simulink model "board_algorithm_2note_length"  (R2023b)
settings: Solver=FixedStepAuto  StartTime=0.0  StopTime=100000.0  RelTol=1e-3
values from neighbouring files (symbols this model uses):
  f_s = 11025    [main.m]
  in_table = single([[0],excitation])    [main.m]
  input = midiMsg_to_input(msgArray)    [main.m]
  N_n = floor(f_s/bps)    [main.m]
  period_sequence_1 = [normalised_period(f_s,input_seq_1(1,:)) ... (first row only)    [main.m]
  period_sequence_2 = [normalised_period(f_s,input_seq_2(1,:)) ... (first row only)    [main.m]
  seq_length = length(input_seq_1)+1    [main.m]
undefined symbols (not defined in the file or in its folder): frac_delay_inter, GPTRIP1SEL, GPTRIP2SEL, TZ1, TZ2
libraries: tiiqmathlib x8, simulink x5, c2837xDlib x3, dspindex x2, c2000lib x1, c280xlib x1, c2802xlib x1
settings Model: ExtModeTrigDuration=8  Creator=andre  LastModifiedBy=Rorya
settings OptimizationCC: DefaultUnderspecifiedDataType=single  EnhancedBackFolding=on  PassReuseOutputArgsAs=Individual arguments  MaxStackSize=1024  OptimizeBlockOrder=speed  DifferentSizesBufferReuse=on  OptimizationCustomize=off  EfficientTunableParamExpr=on
settings DebuggingCC: ParameterTunabilityLossMsg=error
settings HardwareCC: ProdBitPerChar=16  ProdBitPerInt=16  ProdBitPerPointer=32  ProdBitPerSizeT=32  ProdBitPerPtrDiffT=32  ProdLargestAtomicInteger=Integer  ProdLargestAtomicFloat=None  ProdWordSize=16  ProdLongLongMode=on  ProdHWDeviceType=Texas Instruments->C2000  HardwareBoardFeatureSet=SoCBlockset
settings ModelReferenceCC: ModelReferenceNumInstancesAllowed=Single
settings SFSimCC: MATLABDynamicMemAlloc=off
settings RTWCC: Description=Embedded Coder  SystemTargetFile=ert.tlc  HardwareBoard=TI Delfino F28379D LaunchPad  TemplateMakefile=ert_default_tmf  GenerateReport=on  Toolchain=Texas Instruments Code Composer Studio (C2000)  LaunchReport=on  CodeExecutionProfiling=on  CodeProfilingSaveOptions=AllData  CodeProfilingInstrumentation=detailed
settings CodeAppCC: ForceParamTrailComments=on  IgnoreCustomStorageClasses=off  OperatorAnnotations=on  SimulinkDataObjDesc=on  SFDataObjDesc=on  InsertBlockDesc=on
settings ERTTargetCC: CodeReplacementLibrary=TI C28x  ExtModeTransport=4  ExtModeStaticAlloc=on  ExtModeAutomaticAllocSize=off  ExtModeStaticAllocSize=10000  ExtModeMexFile=ext_xcp  ExtModeIntrfLevel=Level2 - Open

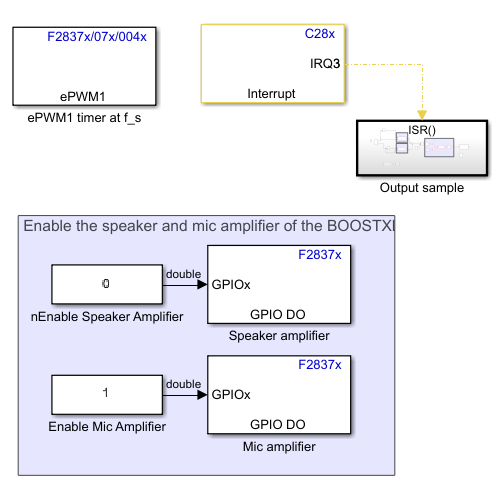
[thumbnail: Simulink's stored preview of the top-level diagram]
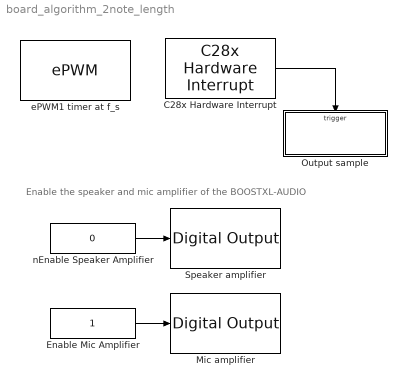
== system board_algorithm_2note_length ==
  note: Enable the speaker and mic amplifier of the BOOSTXL-AUDIO
  C28x Hardware Interrupt : c2000lib/Scheduling/C28x Hardware Interrupt  irqnumbers=[3]  pienumbers=[1]  irqpriorities=[30]  irqpreempts=[1]  showinput=off  dspchiptype=C280X
  Enable Mic Amplifier : Constant
  Mic amplifier : c2837xDlib/Digital Output  GPIO_Number=GPIO96~GPIO103  GPIO_Bit0=off  GPIO_BIT0_Toggle=off  GPIO_Bit1=on  GPIO_BIT1_Toggle=off  GPIO_Bit2=off  GPIO_BIT2_Toggle=off  GPIO_Bit3=off  GPIO_BIT3_Toggle=off  GPIO_Bit4=off  GPIO_BIT4_Toggle=off  GPIO_Bit5=off  GPIO_BIT5_Toggle=off  GPIO_Bit6=off  GPIO_BIT6_Toggle=off  GPIO_Bit7=off  GPIO_BIT7_Toggle=off
  Output sample : Subsystem  TreatAsAtomicUnit=on
  Speaker amplifier : c2837xDlib/Digital Output  GPIO_Number=GPIO24~GPIO31  GPIO_Bit0=off  GPIO_BIT0_Toggle=off  GPIO_Bit1=off  GPIO_BIT1_Toggle=off  GPIO_Bit2=on  GPIO_BIT2_Toggle=off  GPIO_Bit3=off  GPIO_BIT3_Toggle=off  GPIO_Bit4=off  GPIO_BIT4_Toggle=off  GPIO_Bit5=off  GPIO_BIT5_Toggle=off  GPIO_Bit6=off  GPIO_BIT6_Toggle=off  GPIO_Bit7=off  GPIO_BIT7_Toggle=off
  ePWM1 timer at f_s : c2802xlib/ePWM  PwmType=C2000_Type4  useModule=ePWM1  ePWMxLINKTBPRD=Not Linked  periodUnits=Seconds  timerSource=Specify via dialog  timerPeriod_clk=1000  timerPeriod_sec=1/f_s  tbshadow=Counter equals to zero  countingMode=Up  phaseActiveEnable=Set counter to phase value specified via dialog  phaseDirection=Count down after sync  phaseActive=6250  synchronizationEnable=off  dcaevt1Sync=off  dcbevt1Sync=off  synchronizationOption=Disable  dcbevt1SyncOut=off  dcaevt1SyncOut=off  cmpdSyncOut=off  cmpcSyncOut=off  cmpbSyncOut=off  zeroSyncOut=off  swfSyncOut=off  perSynchronizationOption=Counter equals to period (CTR=PRD)  clockPrescale=1  HSclockPrescale=1  enswap=off  ePWMxAStatus=off  ePWMxAactionLogic1=Do nothing  ePWMxAactionLogic2=Do nothing  ePWMxAactionLogic3=Do nothing  ePWMxAactionLogic4=Set  ePWMxAactionLogic5=Do nothing  ePWMxAactionLogic6=Do nothing  ePWMxACSFenable=off  ePWMxACSFvalue=Forcing disable  ePWMxASFreload=Zero  ePWMxBStatus=off  ePWMxBactionLogic1=Set  ePWMxBactionLogic2=Clear  ePWMxBactionLogic3=Do nothing  ePWMxBactionLogic4=Do nothing  ePWMxBactionLogic5=Clear  ePWMxBactionLogic6=Set  ePWMxBCSFenable=off  ePWMxBCSFvalue=Forcing disable  ePWMxBSFreload=Zero  ePWNxBOutWay=off  ePWMxLINKCMPA=Not Linked  CMPAUnits=Percentages  CMPASource=Specify via dialog  CMPAValue_per=50  CMPAValue_clk=50  enCMPAshadow=Counter equals to zero (CTR=Zero)  ePWMxLINKCMPB=Not Linked  CMPBUnits=Clock cycles  CMPBSource=Specify via dialog  CMPBValue_per=50  CMPBValue_clk=32000  enCMPBshadow=Counter equals to zero (CTR=Zero)  ePWMxLINKCMPC=Not Linked  CMPCUnits=Clock cycles  CMPCSource=Specify via dialog  CMPCValue_per=50  CMPCValue_clk=32000  enCMPCshadow=Counter equals to zero (CTR=Zero)  ePWMxLINKCMPD=Not Linked  CMPDUnits=Clock cycles  CMPDSource=Specify via dialog  CMPDValue_per=50  CMPDValue_clk=32000  enCMPDshadow=Counter equals to zero (CTR=Zero)  enableDBePWMxA=off  enableDBePWMxB=off  enhalfcycle=off  DBpolarity=Active high (AH)  DBedgeDelay=Positive  DBSource_ePWMxA=ePWMxA  DBSource_ePWMxB=ePWMxA  DBPeriodUnits=Clock cycles  DBperiodSource=Specify via dialog  REDperiod=0  FEDperiod=0  REDperiod_sec=0  FEDperiod_sec=0  LoadModeDBRED=Immediate without using shadow  LoadModeDBFED=Immediate without using shadow  adcstartModuleA=off  adcrequestEventA=First event  adcstartEventA=Digital Compare Module A Event 1 start of conversion (DCAEVT1.soc)  adcstartEventA_type2=Counter equals to zero (CTR=Zero)  adcstartModuleB=off  adcrequestEventB=First event  adcstartEventB=Counter equals to zero (CTR=Zero)  adcstartEventB_type2=Counter equals to zero (CTR=Zero)  intEn=on  intPrd=First event  intSel=Counter equals to zero (CTR=Zero)  intSel_type2=Counter equals to zero (CTR=Zero)  hrpe=off  enHRPWM=off  HRPWM_LoadMode=Counter equals to period (CTR=PRD)  HRPWM_CTLMode=Duty or Period control mode  HRPWM_EDGMode=Both edge  hrpeb=off  enHRPWMB=off  HRPWM_LoadModeB=Counter equals to zero (CTR=ZERO)  HRPWM_CTLModeB=Duty or Period control mode  HRPWM_EDGModeB=Both edge  enHRDBRED=off  enHRDBFED=off  enSFO=on  enautoconv=on  chopperEnable=off  chopperFrequency=1  chopperFirstwidth=1  chopperDuty=12.5%  tripZonesource=Specify via dialog  tzselOSHT1=off  tzselOSHT2=off  tzselOSHT3=off  tzselOSHDCAEV1=off  tzselOSHDCBEV1=off  tzselCBC1=off  tzselCBC2=off  tzselCBC3=off  tzselCBCDCAEV2=off  tzselCBCDCBEV2=off  tzselOSHT4=off  tzselOSHT5=off  tzselOSHT6=off  tzselCBC4=off  tzselCBC5=off  tzselCBC6=off  enTzOstIntr=off  enTzCbcIntr=off  enTzDCAEVT1Intr=off  enTzDCAEVT2Intr=off  enTzDCBEVT1Intr=off  enTzDCBEVT2Intr=off  ePWMxAforced=No action  ePWMxBforced=No action  DCAEVT1forced=No action  DCBEVT1forced=No action  DCAEVT2forced=No action  DCBEVT2forced=No action  dcah=Trip Zone 1 input (TZ1)  dcal=Trip Zone 2 input (TZ2)  dcbh=Trip Zone 1 input (TZ1)  dcbl=Trip Zone 2 input (TZ2)  dcah_type2=GPTRIP1SEL/(TZ1)  dcal_type2=GPTRIP2SEL/(TZ2)  dcbh_type2=GPTRIP1SEL/(TZ1)  dcbl_type2=GPTRIP2SEL/(TZ2)  gendcaevt1=Event disabled  gendcaevt2=Event disabled  gendcbevt1=Event disabled  gendcbevt2=Event disabled  dcaevt1src=DCAEVT1 with sync  dcaevt2src=DCAEVT2 with sync  dcbevt1src=DCBEVT1 with sync  dcbevt2src=DCBEVT2 with sync  pulsesel=Counter equals to zero (CTR=Zero)  blankinv=off  blankoffset=0  blankwidth=0  evsrcsel=Filtered version of DCAEVT1 (DCAEVT1FILT)  encape=off
  nEnable Speaker Amplifier : Constant  Value=0
  wires:
  Enable Mic Amplifier/1 -> Mic amplifier/1
  nEnable Speaker Amplifier/1 -> Speaker amplifier/1
  C28x Hardware Interrupt/1 -> Output sample/Trigger

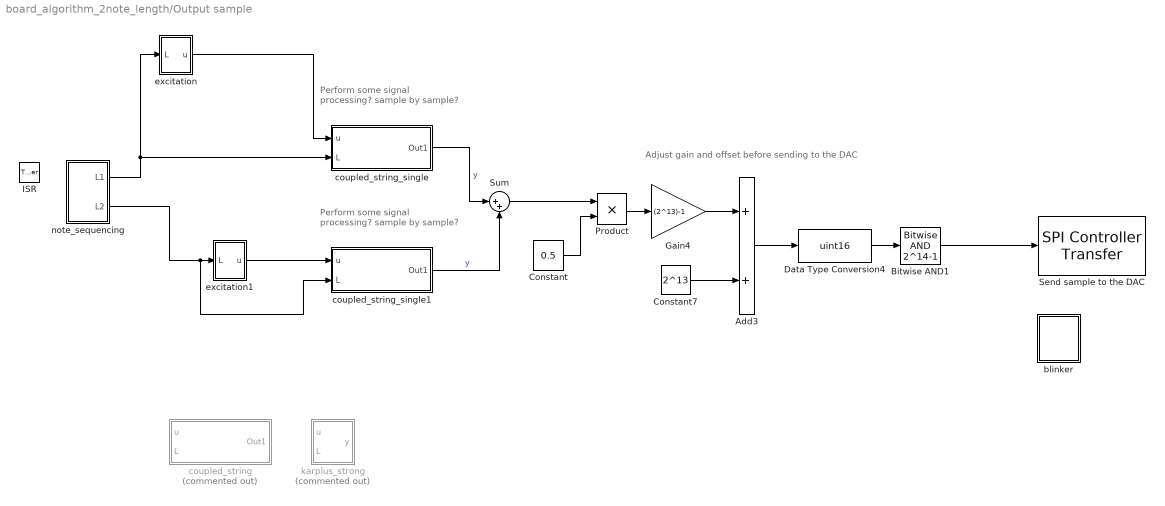
== system board_algorithm_2note_length/Output sample ==
  note: Adjust gain and offset before sending to the DAC
  note: Perform some signal
      | processing?
      | sample by sample?
  note: Perform some signal
      | processing?
      | sample by sample?
  ISR : TriggerPort  TriggerType=function-call  VariantControl=(inherit)
  Add3 : Sum
  Bitwise AND1 : simulink/Logic and Bit Operations/Bitwise Operator  logicop=AND  UseBitMask=on  BitMask=2^14-1  BitMaskRealWorld=Stored Integer
  Constant : Constant  Value=0.5
  Constant7 : Constant  Value=2^13  OutDataTypeStr=single
  Data Type Conversion4 : DataTypeConversion  OutDataTypeStr=uint16  SaturateOnIntegerOverflow=off  RndMeth=Floor
  Gain4 : Gain  Gain=(2^13)-1
  Product : Product
  Send sample to the DAC : c280xlib/SPI Controller Transfer  SPISelect=SPI_B  ClockPolarity=Rising_edge  ClockPhase=Delay_half_cycle  SPIModule=uint32(0)  Mode=Master  BusSpeed=uint32(1000000)  FirstBitToTransfer=Most significant bit (MSB)  ClockMode=0  BlockFunction=Transfer  EnableRegisterAddress=off  RegisterAddress=0  OutputDataType=int8  OutputDataLength=1  DataBits=16  UseCustomSSPin=Explicit GPIO calls  ActiveLowSSPin=Active low  Pin=27
  Sum : Sum  Inputs=|++
  blinker : Subsystem
  coupled_string : Subsystem  Commented=on
  coupled_string_single : Subsystem
  coupled_string_single1 : Subsystem
  excitation : Subsystem
  excitation1 : Subsystem
  karplus_strong : Subsystem  Commented=on
  note_sequencing : Subsystem
  wires:
  Data Type Conversion4/1 -> Bitwise AND1/1
  Gain4/1 -> Add3/1
  Bitwise AND1/1 -> Send sample to the DAC/1
  Add3/1 -> Data Type Conversion4/1
  Constant7/1 -> Add3/2
  coupled_string_single/1(Out1) -> Sum/1  "y"
  coupled_string_single1/1(Out1) -> Sum/2  "y"
  Sum/1 -> Product/1
  Constant/1 -> Product/2
  note_sequencing/2(L2) -> coupled_string_single1/2(L), excitation1/1(L)
  Product/1 -> Gain4/1
  excitation/1(u) -> coupled_string_single/1(u)
  note_sequencing/1(L1) -> coupled_string_single/2(L), excitation/1(L)
  excitation1/1(u) -> coupled_string_single1/1(u)

== system board_algorithm_2note_length/Output sample/blinker ==
  Add : Sum
  Blink LED : c2837xDlib/Digital Output  GPIO_Number=GPIO24~GPIO31  GPIO_Bit0=off  GPIO_BIT0_Toggle=off  GPIO_Bit1=off  GPIO_BIT1_Toggle=off  GPIO_Bit2=off  GPIO_BIT2_Toggle=off  GPIO_Bit3=off  GPIO_BIT3_Toggle=off  GPIO_Bit4=off  GPIO_BIT4_Toggle=off  GPIO_Bit5=off  GPIO_BIT5_Toggle=off  GPIO_Bit6=off  GPIO_BIT6_Toggle=off  GPIO_Bit7=on  GPIO_BIT7_Toggle=on
  Compare To Zero : simulink/Logic and Bit Operations/Compare To Zero  relop===  OutDataTypeStr=uint8
  Constant1 : Constant  OutDataTypeStr=uint16
  Constant2 : Constant  Value=f_s  OutDataTypeStr=uint16
  Mod : Math  Operator=mod
  Unit Delay : UnitDelay  SampleTime=-1  HasFrameUpgradeWarning=on
  wires:
  Compare To Zero/1 -> Blink LED/1
  Mod/1 -> Unit Delay/1, Compare To Zero/1
  Unit Delay/1 -> Add/2
  Add/1 -> Mod/1
  Constant2/1 -> Mod/2
  Constant1/1 -> Add/1

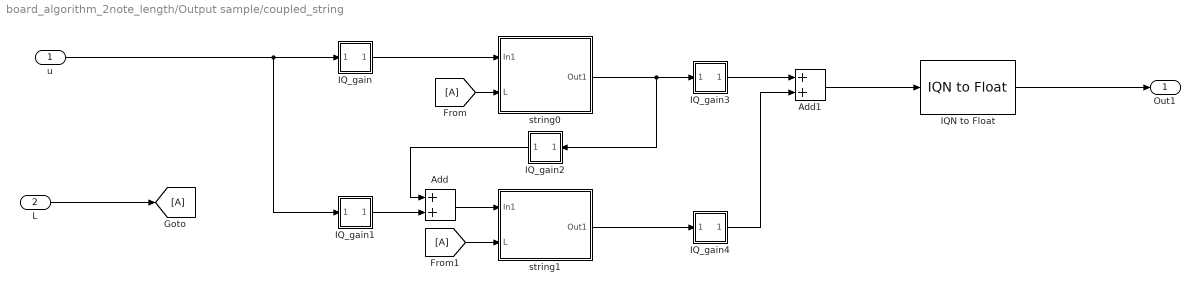
== system board_algorithm_2note_length/Output sample/coupled_string ==
  u : Inport
  L : Inport  Port=2
  Add : Sum  OutDataTypeStr=fixdt(1,32,30)  AccumDataTypeStr=fixdt(1,32,30)
  Add1 : Sum  OutDataTypeStr=Inherit: Same as first input
  From : From
  From1 : From
  Goto : Goto
  IQN to Float : tiiqmathlib/IQN to Float
  IQ_gain : Subsystem
  IQ_gain1 : Subsystem
  IQ_gain2 : Subsystem
  IQ_gain3 : Subsystem
  IQ_gain4 : Subsystem
  string0 : Subsystem
  string1 : Subsystem
  Out1 : Outport
  wires:
  string0/1(Out1) -> IQ_gain3/1(In1), IQ_gain2/1(In1)
  Add/1 -> string1/1(In1)
  IQ_gain/1(Out1) -> string0/1(In1)
  IQ_gain2/1(Out1) -> Add/1
  IQ_gain1/1(Out1) -> Add/2
  string1/1(Out1) -> IQ_gain4/1(In1)
  IQ_gain3/1(Out1) -> Add1/1
  Add1/1 -> IQN to Float/1
  L/1 -> Goto/1
  From/1 -> string0/2(L)
  From1/1 -> string1/2(L)
  IQ_gain4/1(Out1) -> Add1/2
  IQN to Float/1 -> Out1/1
  u/1 -> IQ_gain1/1(In1), IQ_gain/1(In1)

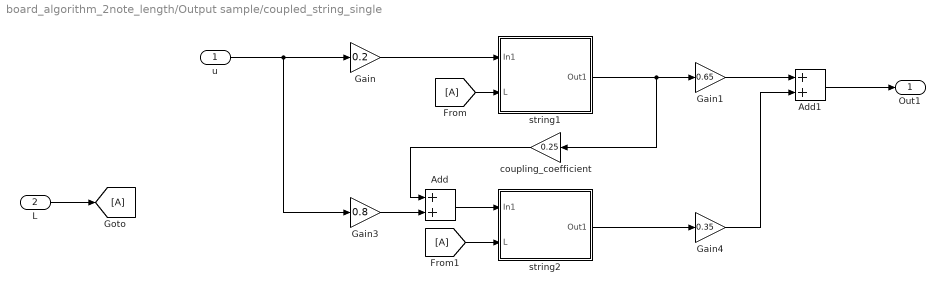
== system board_algorithm_2note_length/Output sample/coupled_string_single ==
  u : Inport  OutDataTypeStr=single
  L : Inport  Port=2
  Add : Sum
  Add1 : Sum
  From : From
  From1 : From
  Gain : Gain  Gain=0.2
  Gain1 : Gain  Gain=0.65
  Gain3 : Gain  Gain=0.8
  Gain4 : Gain  Gain=0.35
  Goto : Goto
  coupling_coefficient : Gain  Gain=0.25
  string1 : Subsystem
  string2 : Subsystem
  Out1 : Outport  OutDataTypeStr=single
  wires:
  string1/1(Out1) -> coupling_coefficient/1, Gain1/1
  Add/1 -> string2/1(In1)
  Gain/1 -> string1/1(In1)
  coupling_coefficient/1 -> Add/1
  Gain3/1 -> Add/2
  string2/1(Out1) -> Gain4/1
  Gain1/1 -> Add1/1
  From/1 -> string1/2(L)
  From1/1 -> string2/2(L)
  Gain4/1 -> Add1/2
  u/1 -> Gain/1, Gain3/1
  L/1 -> Goto/1
  Add1/1 -> Out1/1

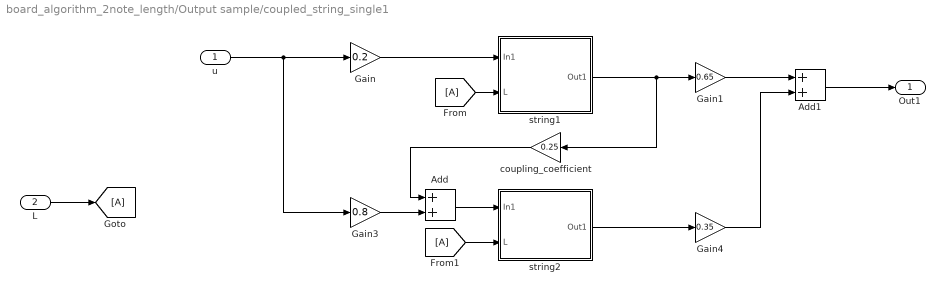
== system board_algorithm_2note_length/Output sample/coupled_string_single1 ==
  u : Inport  OutDataTypeStr=single
  L : Inport  Port=2
  Add : Sum
  Add1 : Sum
  From : From
  From1 : From
  Gain : Gain  Gain=0.2
  Gain1 : Gain  Gain=0.65
  Gain3 : Gain  Gain=0.8
  Gain4 : Gain  Gain=0.35
  Goto : Goto
  coupling_coefficient : Gain  Gain=0.25
  string1 : Subsystem
  string2 : Subsystem
  Out1 : Outport  OutDataTypeStr=single
  wires:
  string1/1(Out1) -> coupling_coefficient/1, Gain1/1
  Add/1 -> string2/1(In1)
  Gain/1 -> string1/1(In1)
  coupling_coefficient/1 -> Add/1
  Gain3/1 -> Add/2
  string2/1(Out1) -> Gain4/1
  Gain1/1 -> Add1/1
  From/1 -> string1/2(L)
  From1/1 -> string2/2(L)
  Gain4/1 -> Add1/2
  u/1 -> Gain/1, Gain3/1
  L/1 -> Goto/1
  Add1/1 -> Out1/1

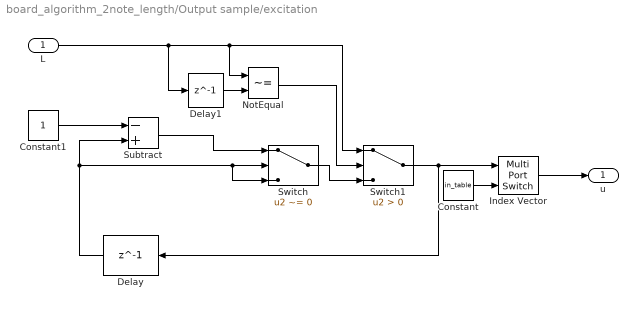
== system board_algorithm_2note_length/Output sample/excitation ==
  L : Inport
  Constant : Constant  Value=in_table  SampleTime=-1
  Constant1 : Constant  SampleTime=-1
  Delay : Delay  DelayLength=1  InitialCondition=0  UseCircularBuffer=on
  Delay1 : Delay  DelayLength=1
  Index Vector : MultiPortSwitch  DataPortOrder=Zero-based contiguous  Inputs=1  zeroidx=on  SaturateOnIntegerOverflow=off  InputSameDT=off
  NotEqual : RelationalOperator  Operator=~=  OutDataTypeStr=boolean  RndMeth=Simplest  InputSameDT=off
  Subtract : Sum  Inputs=-+
  Switch : Switch  Criteria=u2 ~= 0  SaturateOnIntegerOverflow=off  InputSameDT=off
  Switch1 : Switch  Criteria=u2 > Threshold  SaturateOnIntegerOverflow=off  InputSameDT=off
  u : Outport
  wires:
  Constant1/1 -> Subtract/1
  Subtract/1 -> Switch/1
  Switch1/1 -> Index Vector/1, Delay/1
  L/1 -> Delay1/1, NotEqual/1, Switch1/1
  NotEqual/1 -> Switch1/2
  Delay1/1 -> NotEqual/2
  Delay/1 -> Switch/3, Switch/2, Subtract/2
  Switch/1 -> Switch1/3
  Index Vector/1 -> u/1
  Constant/1 -> Index Vector/2

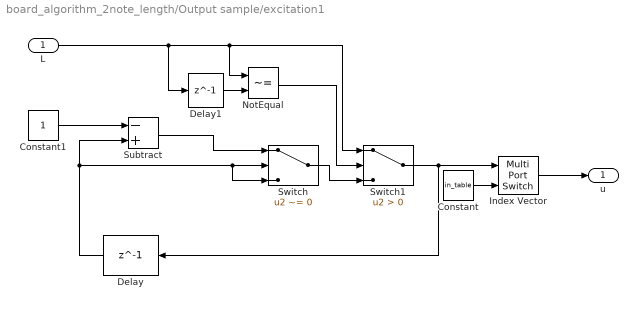
== system board_algorithm_2note_length/Output sample/excitation1 ==
  L : Inport
  Constant : Constant  Value=in_table  SampleTime=-1
  Constant1 : Constant  SampleTime=-1
  Delay : Delay  DelayLength=1  InitialCondition=0  UseCircularBuffer=on
  Delay1 : Delay  DelayLength=1
  Index Vector : MultiPortSwitch  DataPortOrder=Zero-based contiguous  Inputs=1  zeroidx=on  SaturateOnIntegerOverflow=off  InputSameDT=off
  NotEqual : RelationalOperator  Operator=~=  OutDataTypeStr=boolean  RndMeth=Simplest  InputSameDT=off
  Subtract : Sum  Inputs=-+
  Switch : Switch  Criteria=u2 ~= 0  SaturateOnIntegerOverflow=off  InputSameDT=off
  Switch1 : Switch  Criteria=u2 > Threshold  SaturateOnIntegerOverflow=off  InputSameDT=off
  u : Outport
  wires:
  Constant1/1 -> Subtract/1
  Subtract/1 -> Switch/1
  Switch1/1 -> Index Vector/1, Delay/1
  L/1 -> Delay1/1, NotEqual/1, Switch1/1
  NotEqual/1 -> Switch1/2
  Delay1/1 -> NotEqual/2
  Delay/1 -> Switch/3, Switch/2, Subtract/2
  Switch/1 -> Switch1/3
  Index Vector/1 -> u/1
  Constant/1 -> Index Vector/2

== system board_algorithm_2note_length/Output sample/karplus_strong ==
  u : Inport
  L : Inport  Port=2
  Discrete FIR Filter : DiscreteFir
  Sum : Sum  Inputs=|++
  Variable Integer Delay : Delay  DelayLengthSource=Input port  DelayLengthUpperLimit=256  PreventDirectFeedthrough=on  UseCircularBuffer=on
      settings: InputPortMap=u0,p1
  decay constant : Gain
  y : Outport
  wires:
  Variable Integer Delay/1 -> Discrete FIR Filter/1
  L/1 -> Variable Integer Delay/2
  decay constant/1 -> Sum/2
  Sum/1 -> y/1, Variable Integer Delay/1  "y"
  u/1 -> Sum/1
  Discrete FIR Filter/1 -> decay constant/1

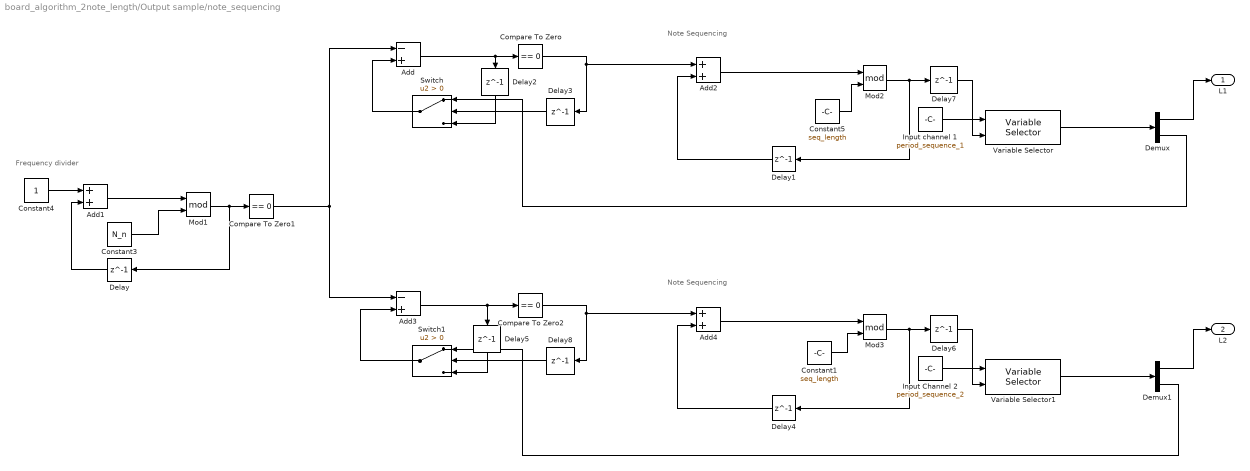
== system board_algorithm_2note_length/Output sample/note_sequencing ==
  note: Frequency divider
  note: Note Sequencing
  note: Note Sequencing
  Add : Sum  Inputs=-+
  Add1 : Sum
  Add2 : Sum
  Add3 : Sum  Inputs=-+
  Add4 : Sum
  Compare To Zero : simulink/Logic and Bit Operations/Compare To Zero  relop===  OutDataTypeStr=boolean
  Compare To Zero1 : simulink/Logic and Bit Operations/Compare To Zero  relop===  OutDataTypeStr=boolean
  Compare To Zero2 : simulink/Logic and Bit Operations/Compare To Zero  relop===  OutDataTypeStr=boolean
  Constant1 : Constant  Value=seq_length  OutDataTypeStr=uint32
  Constant3 : Constant  Value=N_n  OutDataTypeStr=uint32
  Constant4 : Constant  OutDataTypeStr=uint32
  Constant5 : Constant  Value=seq_length  OutDataTypeStr=uint32
  Delay : Delay  DelayLength=1  InitialCondition=0  UseCircularBuffer=on
  Delay1 : Delay  DelayLength=1  InitialCondition=0  UseCircularBuffer=on
  Delay{2..3,5..8} (6 alike) : Delay  DelayLength=1  InitialCondition=0
  Delay4 : Delay  DelayLength=1  InitialCondition=0  UseCircularBuffer=on
  Demux : Demux  Outputs=2
  Demux1 : Demux  Outputs=2
  Input Channel 2 : Constant  Value=period_sequence_2
  Input channel 1 : Constant  Value=period_sequence_1
  Mod1 : Math  Operator=mod
  Mod2 : Math  Operator=mod
  Mod3 : Math  Operator=mod
  Switch : Switch  Criteria=u2 > Threshold  SaturateOnIntegerOverflow=off  InputSameDT=off
  Switch1 : Switch  Criteria=u2 > Threshold  SaturateOnIntegerOverflow=off  InputSameDT=off
  Variable Selector : dspindex/Variable Selector  NumInputs=1  rowsOrCols=Columns  IdxMode=Variable  Elements=[1 3]  ZerOneIdxMode=One-based  errmode=Clip Index  FillMode=on  FillValues=0
  Variable Selector1 : dspindex/Variable Selector  NumInputs=1  rowsOrCols=Columns  IdxMode=Variable  Elements=[1 3]  ZerOneIdxMode=One-based  errmode=Clip Index  FillMode=on  FillValues=0
  L1 : Outport
  L2 : Outport  Port=2
  wires:
  Constant5/1 -> Mod2/2
  Demux/2 -> Switch/1
  Delay/1 -> Add1/2
  Delay1/1 -> Add2/2
  Add2/1 -> Mod2/1
  Compare To Zero/1 -> Delay3/1, Add2/1
  Constant3/1 -> Mod1/2
  Mod1/1 -> Compare To Zero1/1, Delay/1
  Mod2/1 -> Delay7/1, Delay1/1
  Demux/1 -> L1/1
  Add1/1 -> Mod1/1
  Input channel 1/1 -> Variable Selector/1
  Constant4/1 -> Add1/1
  Add/1 -> Compare To Zero/1, Delay2/1
  Add3/1 -> Delay5/1, Compare To Zero2/1
  Input Channel 2/1 -> Variable Selector1/1
  Demux1/1 -> L2/1
  Compare To Zero2/1 -> Delay8/1, Add4/1
  Mod3/1 -> Delay6/1, Delay4/1
  Compare To Zero1/1 -> Add3/1, Add/1
  Delay4/1 -> Add4/2
  Add4/1 -> Mod3/1
  Demux1/2 -> Switch1/1
  Constant1/1 -> Mod3/2
  Delay6/1 -> Variable Selector1/2
  Variable Selector1/1 -> Demux1/1
  Delay7/1 -> Variable Selector/2
  Variable Selector/1 -> Demux/1
  Delay3/1 -> Switch/2
  Delay8/1 -> Switch1/2
  Switch/1 -> Add/2
  Switch1/1 -> Add3/2
  Delay5/1 -> Switch1/3
  Delay2/1 -> Switch/3

== system board_algorithm_2note_length/Output sample/coupled_string/IQ_gain ==
  In1 : Inport  OutDataTypeStr=fixdt(1,32,30)
  Constant : Constant  Value=0.2  OutDataTypeStr=fixdt(1,32,30)
  IQN x IQN : tiiqmathlib/IQN x IQN  multiplyOption=Multiply
  Out1 : Outport  OutDataTypeStr=fixdt(1,32,30)
  wires:
  In1/1 -> IQN x IQN/1
  IQN x IQN/1 -> Out1/1
  Constant/1 -> IQN x IQN/2

== system board_algorithm_2note_length/Output sample/coupled_string/IQ_gain1 ==
  In1 : Inport
  Constant : Constant  Value=0.8  OutDataTypeStr=fixdt(1,32,30)
  IQN x IQN : tiiqmathlib/IQN x IQN  multiplyOption=Multiply
  Out1 : Outport
  wires:
  In1/1 -> IQN x IQN/1
  IQN x IQN/1 -> Out1/1
  Constant/1 -> IQN x IQN/2

== system board_algorithm_2note_length/Output sample/coupled_string/IQ_gain2 ==
  In1 : Inport  OutDataTypeStr=fixdt(1,32,30)  LockScale=on
  Constant : Constant  Value=0.25  OutDataTypeStr=fixdt(1,32,30)
  IQN x IQN : tiiqmathlib/IQN x IQN  multiplyOption=Multiply
  Out1 : Outport  OutDataTypeStr=fixdt(1,32,30)
  wires:
  In1/1 -> IQN x IQN/1
  IQN x IQN/1 -> Out1/1
  Constant/1 -> IQN x IQN/2

== system board_algorithm_2note_length/Output sample/coupled_string/IQ_gain3 ==
  In1 : Inport
  Constant : Constant  Value=0.65  OutDataTypeStr=fixdt(1,32,30)
  IQN x IQN : tiiqmathlib/IQN x IQN  multiplyOption=Multiply
  Out1 : Outport
  wires:
  In1/1 -> IQN x IQN/1
  IQN x IQN/1 -> Out1/1
  Constant/1 -> IQN x IQN/2

== system board_algorithm_2note_length/Output sample/coupled_string/IQ_gain4 ==
  In1 : Inport
  Constant : Constant  Value=0.35  OutDataTypeStr=fixdt(1,32,30)
  IQN x IQN : tiiqmathlib/IQN x IQN  multiplyOption=Multiply
  Out1 : Outport
  wires:
  In1/1 -> IQN x IQN/1
  IQN x IQN/1 -> Out1/1
  Constant/1 -> IQN x IQN/2

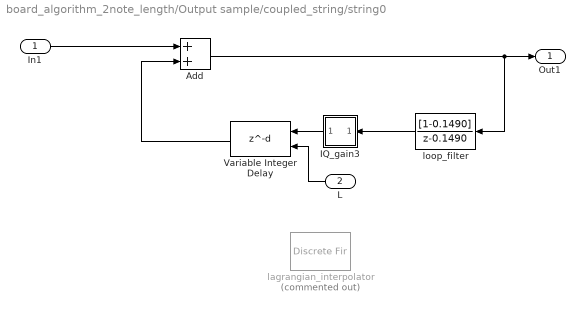
== system board_algorithm_2note_length/Output sample/coupled_string/string0 ==
  In1 : Inport
  L : Inport  Port=2
  Add : Sum  OutDataTypeStr=fixdt(1,32,30)  AccumDataTypeStr=fixdt(1,32,30)
  IQ_gain3 : Subsystem
  Variable Integer Delay : Delay  DelayLengthSource=Input port  DelayLengthUpperLimit=256  PreventDirectFeedthrough=on  UseCircularBuffer=on
      settings: InputPortMap=u0,p1
  lagrangian_interpolator : DiscreteFir  Commented=on  Coefficients=frac_delay_inter
  loop_filter : DiscreteTransferFcn  Numerator=[1-0.1490]  Denominator=[1 -0.1490]  StateDataTypeStr=fixdt(1,32,30)  NumCoefDataTypeStr=fixdt(1,32,30)  DenCoefDataTypeStr=fixdt(1,32,30)  NumProductDataTypeStr=fixdt(1,32,30)  DenProductDataTypeStr=fixdt(1,32,30)  NumAccumDataTypeStr=fixdt(1,32,30)  DenAccumDataTypeStr=fixdt(1,32,30)  OutDataTypeStr=fixdt(1,32,30)
  Out1 : Outport
  wires:
  Add/1 -> loop_filter/1, Out1/1
  loop_filter/1 -> IQ_gain3/1(In1)
  In1/1 -> Add/1
  L/1 -> Variable Integer Delay/2
  IQ_gain3/1(Out1) -> Variable Integer Delay/1
  Variable Integer Delay/1 -> Add/2

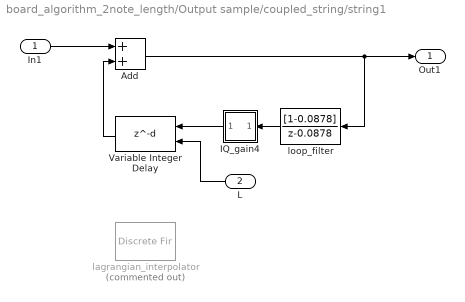
== system board_algorithm_2note_length/Output sample/coupled_string/string1 ==
  In1 : Inport
  L : Inport  Port=2
  Add : Sum  OutDataTypeStr=fixdt(1,32,30)  AccumDataTypeStr=fixdt(1,32,30)
  IQ_gain4 : Subsystem
  Variable Integer Delay : Delay  DelayLengthSource=Input port  DelayLengthUpperLimit=256  PreventDirectFeedthrough=on  UseCircularBuffer=on
      settings: InputPortMap=u0,p1
  lagrangian_interpolator : DiscreteFir  Commented=on  Coefficients=frac_delay_inter
  loop_filter : DiscreteTransferFcn  Numerator=[1-0.0878]  Denominator=[1 -0.0878]  StateDataTypeStr=fixdt(1,32,30)  NumCoefDataTypeStr=fixdt(1,32,30)  DenCoefDataTypeStr=fixdt(1,32,30)  NumProductDataTypeStr=fixdt(1,32,30)  DenProductDataTypeStr=fixdt(1,32,30)  NumAccumDataTypeStr=fixdt(1,32,30)  DenAccumDataTypeStr=fixdt(1,32,30)  OutDataTypeStr=fixdt(1,32,30)
  Out1 : Outport
  wires:
  Add/1 -> loop_filter/1, Out1/1
  loop_filter/1 -> IQ_gain4/1(In1)
  In1/1 -> Add/1
  L/1 -> Variable Integer Delay/2
  Variable Integer Delay/1 -> Add/2
  IQ_gain4/1(Out1) -> Variable Integer Delay/1

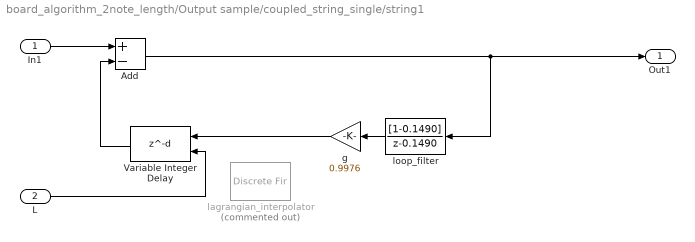
== system board_algorithm_2note_length/Output sample/coupled_string_single/string1 ==
  In1 : Inport
  L : Inport  Port=2
  Add : Sum  Inputs=+-  OutDataTypeStr=single
  Variable Integer Delay : Delay  DelayLengthSource=Input port  DelayLengthUpperLimit=256  PreventDirectFeedthrough=on  UseCircularBuffer=on
      settings: InputPortMap=u0,p1
  g : Gain  Gain=0.9976
  lagrangian_interpolator : DiscreteFir  Commented=on  Coefficients=frac_delay_inter
  loop_filter : DiscreteTransferFcn  Numerator=[1-0.1490]  Denominator=[1 -0.1490]
  Out1 : Outport
  wires:
  Add/1 -> Out1/1, loop_filter/1
  loop_filter/1 -> g/1
  Variable Integer Delay/1 -> Add/2
  In1/1 -> Add/1
  L/1 -> Variable Integer Delay/2
  g/1 -> Variable Integer Delay/1

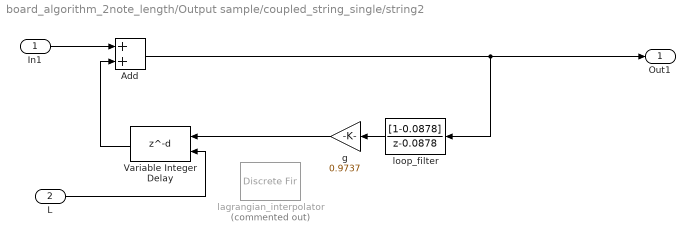
== system board_algorithm_2note_length/Output sample/coupled_string_single/string2 ==
  In1 : Inport
  L : Inport  Port=2
  Add : Sum  OutDataTypeStr=single
  Variable Integer Delay : Delay  DelayLengthSource=Input port  DelayLengthUpperLimit=256  PreventDirectFeedthrough=on  UseCircularBuffer=on
      settings: InputPortMap=u0,p1
  g : Gain  Gain=0.9737
  lagrangian_interpolator : DiscreteFir  Commented=on  Coefficients=frac_delay_inter
  loop_filter : DiscreteTransferFcn  Numerator=[1-0.0878]  Denominator=[1 -0.0878]
  Out1 : Outport
  wires:
  Add/1 -> Out1/1, loop_filter/1
  loop_filter/1 -> g/1
  Variable Integer Delay/1 -> Add/2
  In1/1 -> Add/1
  L/1 -> Variable Integer Delay/2
  g/1 -> Variable Integer Delay/1

== system board_algorithm_2note_length/Output sample/coupled_string_single1/string1 ==
  In1 : Inport
  L : Inport  Port=2
  Add : Sum  Inputs=+-  OutDataTypeStr=single
  Variable Integer Delay : Delay  DelayLengthSource=Input port  DelayLengthUpperLimit=256  PreventDirectFeedthrough=on  UseCircularBuffer=on
      settings: InputPortMap=u0,p1
  g : Gain  Gain=0.9976
  lagrangian_interpolator : DiscreteFir  Commented=on  Coefficients=frac_delay_inter
  loop_filter : DiscreteTransferFcn  Numerator=[1-0.1490]  Denominator=[1 -0.1490]
  Out1 : Outport
  wires:
  Add/1 -> Out1/1, loop_filter/1
  loop_filter/1 -> g/1
  Variable Integer Delay/1 -> Add/2
  In1/1 -> Add/1
  L/1 -> Variable Integer Delay/2
  g/1 -> Variable Integer Delay/1

== system board_algorithm_2note_length/Output sample/coupled_string_single1/string2 ==
  In1 : Inport
  L : Inport  Port=2
  Add : Sum  OutDataTypeStr=single
  Variable Integer Delay : Delay  DelayLengthSource=Input port  DelayLengthUpperLimit=256  PreventDirectFeedthrough=on  UseCircularBuffer=on
      settings: InputPortMap=u0,p1
  g : Gain  Gain=0.9737
  lagrangian_interpolator : DiscreteFir  Commented=on  Coefficients=frac_delay_inter
  loop_filter : DiscreteTransferFcn  Numerator=[1-0.0878]  Denominator=[1 -0.0878]
  Out1 : Outport
  wires:
  Add/1 -> Out1/1, loop_filter/1
  loop_filter/1 -> g/1
  Variable Integer Delay/1 -> Add/2
  In1/1 -> Add/1
  L/1 -> Variable Integer Delay/2
  g/1 -> Variable Integer Delay/1

== system board_algorithm_2note_length/Output sample/coupled_string/string0/IQ_gain3 ==
  In1 : Inport  OutDataTypeStr=fixdt(1,32,30)
  Constant : Constant  Value=0.9976  OutDataTypeStr=fixdt(1,32,30)
  IQN x IQN : tiiqmathlib/IQN x IQN  multiplyOption=Multiply
  Out1 : Outport  OutDataTypeStr=fixdt(1,32,30)
  wires:
  In1/1 -> IQN x IQN/1
  IQN x IQN/1 -> Out1/1
  Constant/1 -> IQN x IQN/2

== system board_algorithm_2note_length/Output sample/coupled_string/string1/IQ_gain4 ==
  In1 : Inport
  Constant : Constant  Value=0.9737  OutDataTypeStr=fixdt(1,32,30)
  IQN x IQN : tiiqmathlib/IQN x IQN  multiplyOption=Multiply
  Out1 : Outport
  wires:
  In1/1 -> IQN x IQN/1
  IQN x IQN/1 -> Out1/1
  Constant/1 -> IQN x IQN/2
